simulink library "PostLimiterEqBtc"  (R2022b)
settings: Solver=VariableStepAuto  StartTime=0.0  StopTime=10.0  RelTol=1e-3
undefined symbols (not defined in the file or in its folder): Config
libraries: FeaturePath x1, RTC x1, HandyTextFile x1, Ann1Path x1, PoolIir x1
settings Model: Creator=kl13806  LastModifiedBy=st51187
settings SolverCC: AlgebraicLoopSolver=TrustRegion
settings DebuggingCC: UnconnectedInputMsg=warning  UnconnectedOutputMsg=warning  UnconnectedLineMsg=warning  SFMachineParentedDataDiag=warning
settings ModelReferenceCC: EnableRefExpFcnMdlSchedulingChecks=on
settings RTWCC: DLArmComputeVersion=19.05

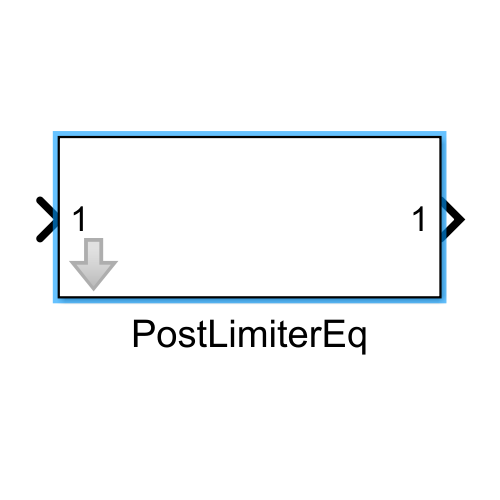
[thumbnail: Simulink's stored preview of the top-level diagram]
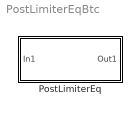
== system PostLimiterEqBtc ==
  PostLimiterEq : Subsystem  mask(Blocklib PostLimiterEq){Config=Config.PostLimiterEq, FeatureName=PostLimiterEq}
      mask prompts: Config "PostLimiterEqConfig"; FeatureName "Feature path name:"
      mask help: This block is an extension of the PoolIIR with Non-Trivial Translations block (aka PoolIirTunable), with the added benefit of an embedded RTC that can switch the filtering process on or off.
      mask init:
      | blkh=gcbh;
      | Config=BTConfig.Assert(blkh,Config);
      | BTConfig.InitSetFeatureIfPresent(blkh,'FeatureName');
      | Config.Validate();
      | 
      | theDsms = {'DisableEq'};
      | CscUtil.SetupDsmsForStaticInit(blkh,theDsms);
      mask Callback Config: BTConfig.CallbackHideIfPresent(gcbh,{'FeatureName'});
      mask TypeOptions FeatureName: Control/FeaturePath/FeatureName | PoolIirTunable/FeatureName

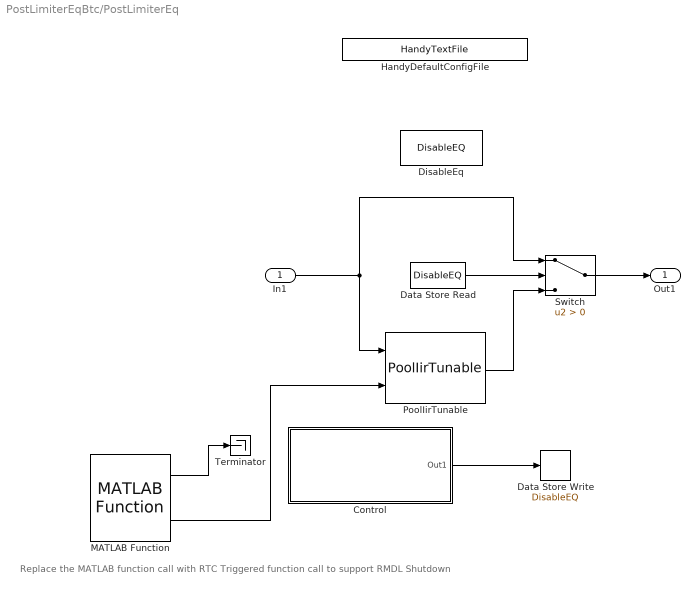
== system PostLimiterEqBtc/PostLimiterEq ==
  note: Replace the MATLAB function call with RTC Triggered function call to support RMDL Shutdown
  In1 : Inport
  Control : Subsystem
  Data Store Read : DataStoreRead  DataStoreName=DisableEQ  IndexOptions=Index vector (dialog)  Indices=1  OutputSizes=1
  Data Store Write : DataStoreWrite  DataStoreName=DisableEQ  IndexOptions=Index vector (dialog)  Indices=1  OutputSizes=1
  DisableEq : DataStoreMemory  DataStoreName=DisableEQ  ReadBeforeWriteMsg=warning  WriteAfterWriteMsg=warning  WriteAfterReadMsg=warning  ShowAdditionalParam=off
  HandyDefaultConfigFile : HandyTextFile/HandyTextFile  TemplateSource=Config  FileSuffix=Init  OpenDialogOnLoad=off  UseThisBlockName=off  AddGrandParentNamePrefix=off  TheDefaultText=|  ShowInLibBrowser=on
      | % $(FILENAME) Setup model parameters for each "Init" callback (e.g. update diagram)
      | sample_rate_in_hertz = 44100;
      | frame_size = 32;
      | sysin_channel_count = 2;
      settings: SourceProductName=Bose Talaria
  MATLAB Function : Ann1Path/Ann1path/MATLAB Function  SystemSampleTime=-1  VariantActivationTime=update diagram  Latency=0  AutoFrameSizeCalculation=off
      settings: LibrarySourceBlock=|
      | simulink/User-Defined
      | Functions/MATLAB Function
  PoolIirTunable : PoolIir/PoolIirTunable  FeatureName=PostLimiterEq  Config=Config
  Switch : Switch  Criteria=u2 > Threshold  SaturateOnIntegerOverflow=off  InputSameDT=off
  Terminator : Terminator
  Out1 : Outport
  wires:
  MATLAB Function/1 -> Terminator/1
  MATLAB Function/2 -> PoolIirTunable/2
  PoolIirTunable/1 -> Switch/3
  Data Store Read/1 -> Switch/2
  Switch/1 -> Out1/1
  In1/1 -> PoolIirTunable/1, Switch/1
  Control/1(Out1) -> Data Store Write/1

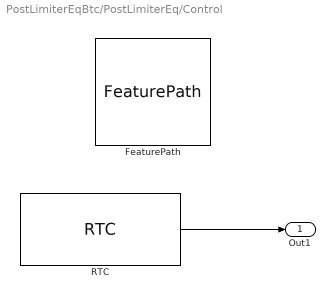
== system PostLimiterEqBtc/PostLimiterEq/Control ==
  FeaturePath : FeaturePath/FeaturePath  FeatureName=PostLimiterEq  IsGroup=off  GroupNumber=-1  IsModule=off  TriggerInit=[95 -131 210 -24]
      settings: SourceProductName=Bose Talaria
  RTC : RTC/RTC  REQ_Priority=RTC_Mask.NormalPriority  RequestAtInit=off  EnableRequest=off  REQElemName1=disableMsg  REQElemType1=int32  REQElemWidth1=1  REQElemInitial1=0  REQElemType2=uint32  REQElemWidth2=1  REQElemInitial2=[]  REQElemType3=uint32  REQElemWidth3=1  REQElemInitial3=[]  REQElemType4=uint32  REQElemWidth4=1  REQElemInitial4=[]  REQElemType5=uint32  REQElemWidth5=1  REQElemInitial5=[]  REQElemType6=uint32  REQElemWidth6=1  REQElemInitial6=[]  REQElemType7=uint32  REQElemWidth7=1  REQElemInitial7=[]  REQElemType8=uint32  REQElemWidth8=1  REQElemInitial8=[]  REQElemType9=uint32  REQElemWidth9=1  REQElemInitial9=[]  REQElemType10=uint32  REQElemWidth10=1  REQElemInitial10=[]  EnableResponse=on  EnableRSP_StatusIn=off  RSPElemType1=uint32  RSPElemWidth1=1  RSPElemType2=uint32  RSPElemWidth2=1  RSPElemType3=uint32  RSPElemWidth3=1  RSPElemType4=uint32  RSPElemWidth4=1  RSPElemType5=uint32  RSPElemWidth5=1  RSPElemType6=uint32  RSPElemWidth6=1  RSPElemType7=uint32  RSPElemWidth7=1  RSPElemType8=uint32  RSPElemWidth8=1  RSPElemType9=uint32  RSPElemWidth9=1  RSPElemType10=uint32  RSPElemWidth10=1  EnableNotification=off  EnableNTF_PrepTrig=off  NTFElemType1=uint32  NTFElemWidth1=1  NTFElemType2=uint32  NTFElemWidth2=1  NTFElemType3=uint32  NTFElemWidth3=1  NTFElemType4=uint32  NTFElemWidth4=1  NTFElemType5=uint32  NTFElemWidth5=1  NTFElemType6=uint32  NTFElemWidth6=1  NTFElemType7=uint32  NTFElemWidth7=1  NTFElemType8=uint32  NTFElemWidth8=1  NTFElemType9=uint32  NTFElemWidth9=1  NTFElemType10=uint32  NTFElemWidth10=1  MaskMessageName=Disable
      settings: SourceProductName=Bose Talaria
  Out1 : Outport
  wires:
  RTC/1 -> Out1/1
